simulink model "insulin_RL"  (R2018a)
settings: Solver=FixedStepAuto  StartTime=0.0  StopTime=100  RelTol=1e-3  AbsTol=1e-5
model workspace (MATLAB code in the model file):
  | load sldemo_autotrans_data; %load initial conditions and other necessary data
libraries: S_TaLiRo x1
Description:
  | Modeling an Automatic Transmission Controller
  | 
  | In this example, Simulink(R) is used to model an automotive drivetrain. Stateflow(R)
  | enhances the Simulink model with its representation of the transmission
  | control logic. Simulink provides a powerful environment for the modeling and
  | simulation of dynamic systems and processes. In many systems, though,
  | supervisory functions like changing modes or invoking new gain schedules must
  | respond to events that may occur and conditions that develop over time. As a
  | result, the environment requires a language capable of managing these multiple
  | modes and developing conditions. In the following example, Stateflow
  | demonstrates its strength in this capacity by performing the function of gear
  | selection in an automatic transmission. This function is combined with the
  | drivetrain dynamics in a natural and intuitive manner by incorporating a
  | Stateflow block in the Simulink block diagram.
settings Model: DataTypeOverride=Double  MinMaxOverflowLogging=ForceOff  ExtModeTrigMode=oneshot  ExtModeArmWhenConnect=off  ExtModeAutoUpdateStatusClock=off  Creator=The MathWorks Inc.  LastModifiedBy=shenhai
settings SolverCC: AutoScaleAbsTol=off  SolverJacobianMethodControl=SparsePerturbation
settings DataIOCC: SaveState=on  SignalLoggingName=sldemo_autotrans_output
settings OptimizationCC: BlockReduction=off  BooleanDataType=off  ExpressionDepthLimit=2147483647  InitFltsAndDblsToZero=on  LifeSpan=inf
settings DebuggingCC: SaveWithParameterizedLinksMsg=none  UnderspecifiedInitializationDetection=Classic  MergeDetectMultiDrivingBlocksExec=none  CheckExecutionContextPreStartOutputMsg=on  CheckExecutionContextRuntimeOutputMsg=on  SignalResolutionControl=TryResolveAllWithWarning  MaxConsecutiveZCsMsg=none  MultiTaskDSMMsg=warning  MultiTaskCondExecSysMsg=none  SigSpecEnsureSampleTimeMsg=none  IntegerOverflowMsg=none  FcnCallInpInsideContextMsg=warning  StateNameClashWarn=warning  InitInArrayFormatMsg=none  SFUnexpectedBacktrackingDiag=warning  SFNoUnconditionalDefaultTransitionDiag=warning  SFExecutionAtInitializationDiag=none  IntegerSaturationMsg=none
settings HardwareCC: ProdBitPerPointer=32  ProdBitPerSizeT=32  ProdBitPerPtrDiffT=32  ProdLargestAtomicFloat=None  ProdIntDivRoundTo=Undefined  ProdEndianess=Unspecified  ProdWordSize=32  ProdHWDeviceType=32-bit Generic
settings ModelReferenceCC: ModelReferenceMinAlgLoopOccurrences=on  PropagateSignalLabelsOutOfModel=off
settings SFSimCC: SFSimEcho=off  SimParseCustomCode=off
settings CodeAppCC: StateflowObjectComments=on
settings GRTTargetCC: TargetFcnLib=ansi_tfl_tmw.mat  TargetLangStandard=C89/C90 (ANSI)  GeneratePreprocessorConditionals=Disable all  CombineOutputUpdateFcns=off  GRTInterface=on
settings ConfigComp: CovMetricSettings=dcmtr  CovHtmlReporting=on  CovSaveCumulativeToWorkspaceVar=on  CovSaveSingleToWorkspaceVar=on  CovExternalEMLEnable=off

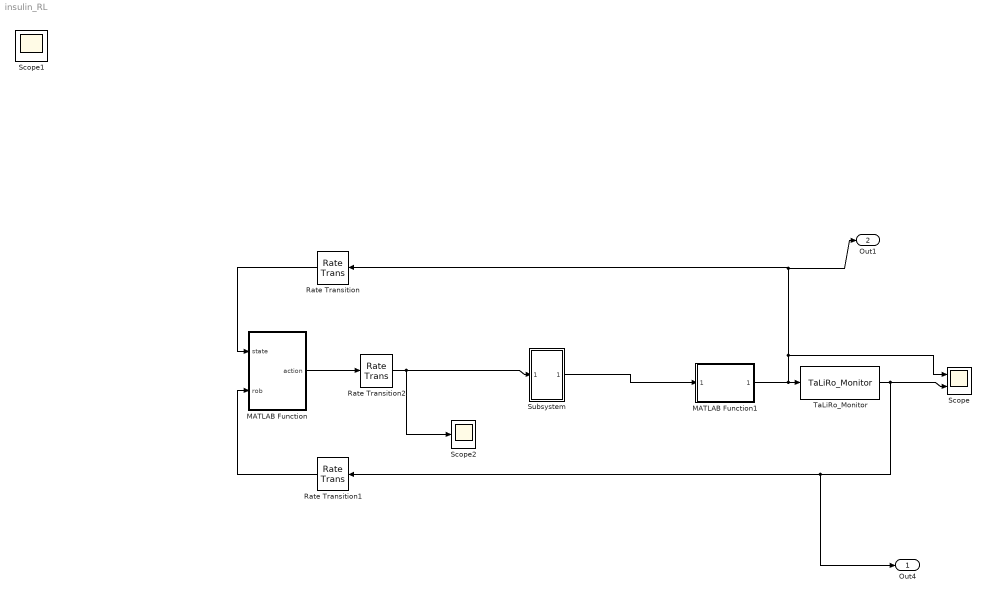
== system insulin_RL ==
  MATLAB Function : MATLAB Function  TreatAsAtomicUnit=on  SystemSampleTime=5
  MATLAB Function1 : MATLAB Function  TreatAsAtomicUnit=on
  Rate Transition : RateTransition  OutPortSampleTimeOpt=Inherit
  Rate Transition1 : RateTransition  InitialCondition=1.5  OutPortSampleTimeOpt=Inherit
  Rate Transition2 : RateTransition  InitialCondition=[40,30,200,40,200,40,35,200,45,0]  OutPortSampleTimeOpt=Inherit
  Scope : Scope  NumInputPorts=2
  Scope2 : Scope
  Subsystem : ModelReference  ModelNameDialog=insulinGlucoseSimHumanCtrl  SimulationMode=Normal  ModelReferenceVersion=1.338
  TaLiRo_Monitor : S_TaLiRo/TaLiRo_Monitor  sample=0.04  specnm=Phi  predmp=Pred
      settings: SourceProductName=S-TaLiRo
  Out4 : Outport
  Out1 : Outport  Port=2  SampleTime=0.04
  Scope1 : Scope
  wires:
  TaLiRo_Monitor/1 -> Scope/2, Rate Transition1/1, Out4/1
  Subsystem/1 -> MATLAB Function1/1(unnormalized)
  Rate Transition/1 -> MATLAB Function/1(state)
  Rate Transition1/1 -> MATLAB Function/2(rob)
  MATLAB Function1/1(normalized) -> Rate Transition/1, Out1/1, Scope/1, TaLiRo_Monitor/1
  Rate Transition2/1 -> Scope2/1, Subsystem/1
  MATLAB Function/1(action) -> Rate Transition2/1

== matlab function insulin_RL/MATLAB Function1 ==
  data: unnormalized input; normalized output
function normalized = normalize(unnormalized)
coder.extrinsic('evalin')
output_range = [0 0; 0 0; 0 0];
output_range = evalin('base', 'output_range');
lower = output_range(:,1);
upper = output_range(:,2);
middle = (lower + upper)/2;
d = (upper - lower)/2;
normalized = (unnormalized - middle) ./ d;

== matlab function insulin_RL/MATLAB Function ==
  data: state input; rob input; action output
function action  = driver(state, rob)
coder.extrinsic('py.driver.driver', 'evalin')
%#codegen
agent = evalin('base', 'agent');
action_normalized = [0 0 0 0 0 0 0 0 0 0];
input_range = [0 0;0 0;0 0;0 0;0 0;0 0;0 0;0 0;0 0;0 0;];
input_range = evalin('base', 'input_range');
action_normalized = double(py.driver.driver(agent, state', rob(1)));
action_normalized = transpose(min([1 1 1 1 1 1 1 1 1 1], max([-1 -1 -1 -1 -1 -1 -1 -1 -1 -1], action_normalized)));
lower = input_range(:,1);
upper = input_range(:,2);
middle = (lower + upper)/2;
action = action_normalized .* (upper - middle) + middle;
